simulink subsystem "ex_modeling_mechanical_system"  (R2019b)
settings: Solver=VariableStepAuto  StartTime=0.0  StopTime=10.0  RelTol=1e-3
PreLoadFcn:
  | addpath(fullfile(matlabroot,'examples','simulink','main'));
  | 
  | ex_modeling_data_mechanical_system
  | 
  | rmpath(fullfile(matlabroot,'examples','simulink','main'));
settings Model: Creator=The MathWorks, Inc.  LastModifiedBy=The MathWorks, Inc.

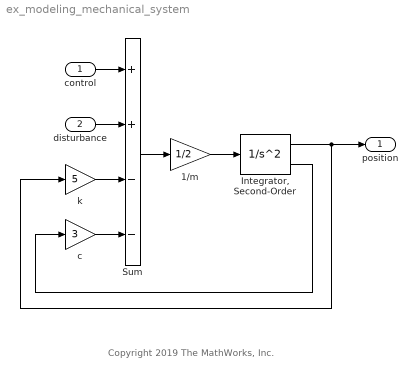
== system ex_modeling_mechanical_system ==
  note: Copyright 2019 The MathWorks, Inc.
  control : Inport
  disturbance : Inport  Port=2
  1/m : Gain  Gain=1/2
  "Integrator, Second-Order" : SecondOrderIntegrator
  Sum : Sum  Inputs=++--
  c : Gain  Gain=3
  k : Gain  Gain=5
  position : Outport  VectorParamsAs1DForOutWhenUnconnected=off
  wires:
  "Integrator, Second-Order"/2 -> c/1
  1/m/1 -> "Integrator, Second-Order"/1
  disturbance/1 -> Sum/2
  Sum/1 -> 1/m/1
  c/1 -> Sum/4
  control/1 -> Sum/1
  "Integrator, Second-Order"/1 -> position/1, k/1
  k/1 -> Sum/3
